simulink model "helicopter_sim"  (R2024b)
settings: Solver=ode4  StartTime=0.0  StopTime=30  FixedStep=ST  RelTol=1e-3
StopFcn:
  | % main rotor flapping restraint
  | if over_flap
  |     warning('MyModel:flapping', '<strong> main rotor blade flapping exceeded limits </strong>');
  | end
  | % tail rotor flapping restraint
  | if over_flap_tr
  |     warning('MyModel:flapping_tr', '<strong> tail rotor blade flapping exceeded limits </strong>');
  | end
  | % main rotor load limit
  | if load_mr
  |     warning('MyModel:load_mr', '<strong> main rotor load limit reached </strong>');
  | end
  | % main rotor power limit
  | if power_mr
  |     warning('MyModel:power_mr', '<strong> transmission maximum power rating reached </strong>');
  | end
  | % main rotor blade stall
  | if stall_mr
  |     warning('MyModel:blade_stall', '<strong> main rotor blade stall </strong>');
  | end
  | clear over_flap over_flap_tr load_mr power_mr stall_mr
values from neighbouring files (symbols this model uses):
  a_0 = [ 0 0 0 ]'*pi/180    [parameters.m]    (also in trim.m = [ flap_ss(1) flap_ss(2) flap_ss(3) ]')
  a_hs = 6    [parameters.m]
  a_vs = 6    [parameters.m]
  AKBETA = 0    [parameters.m]
  AKONE = 0    [parameters.m]
  AKONETR = tan(30*(pi/180))    [parameters.m]
  alpha_stall = 15    [parameters.m]
  AOP = 0    [parameters.m]
  AOPTR = 0    [parameters.m]
  AR_hs = 4.5    [parameters.m]
  AR_vs = 1.8    [parameters.m]
  ASLOPE = 6    [parameters.m]
  ASLOPETR = 6    [parameters.m]
  BLADES = 4    [parameters.m]
  BLADESTR = 3    [parameters.m]
  BLCG = 0    [parameters.m]
  BLHS = 0    [parameters.m]
  BLMR = 0    [parameters.m]
  BLRPF = 0    [parameters.m]
  BLTR = -1.8*Ft_m    (= -0.54864)    [parameters.m]
  BLVS = 0    [parameters.m]
  CD_f = [1.774 0.2043 7]    [parameters.m]
  CD_mr = [0.0107 -0.151 1.72]    [parameters.m]
  CD_tr = [ 0.0107 -0.151 1.72 ]    [parameters.m]
  chi_mr = 1    [parameters.m]
  chi_tr = 1    [parameters.m]
  CHORD = 2*Ft_m    (= 0.6096)    [parameters.m]
  CHORDTR = 1*Ft_m    (= 0.3048)    [parameters.m]
  CL_f = [-0.4279 10.33]    [parameters.m]
  CL_max_hs = 1.2    [parameters.m]
  CL_max_vs = 1.2    [parameters.m]
  CLL_f = [0.0696 6.336]    [parameters.m]
  CM_f = [-4.4961 49.522]    [parameters.m]
  CN_f = [0.0396 -21.699]    [parameters.m]
  CY_f = [-0.0359 -16.987]    [parameters.m]
  D = zeros(9,4)    [linearization.m]
  dyn_viscosity = 17.89e-6    (= 1.789e-05)    [parameters.m]
  e_hs = 0.8    [parameters.m]
  e_vs = 0.8    [parameters.m]
  EPSLN = 0.05    [parameters.m]
  euler0 = [ 0 0 0 ]'*pi/180    [parameters.m]    (also in trim.m = [ euler_trim(1)*abs(max_att) euler_trim(2)*abs(max_att) eule)
  fc = [  100*Kn_mps ... (first row only)    [parameters.m]
  GAMMA = 8.1    [parameters.m]
  GAMMATR = 4    [parameters.m]
  href = 0    [parameters.m]
  i_hs = -3*(pi/180)+a0_hs    (= -0.0523598775598)    [parameters.m]
  i_s = 0    [parameters.m]
  i_vs = 0*(pi/180)+a0_vs    (= -0.0872664625997)    [parameters.m]
  Jbeta = 1/3*m_blade*ROTOR^3*(1-EPSLN)^3    (= 3891.86391298)    [parameters.m]
  k_ind = 1    [parameters.m]
  k_ind_tr = 1    [parameters.m]
  kv_tr = 0.8    [parameters.m]
  Lambda_hs = 13*(pi/180)    (= 0.226892802759)    [parameters.m]
  Lambda_vs = 27*(pi/180)    (= 0.471238898038)    [parameters.m]
  lat_cyc_range = [ -15 15 ]    [parameters.m]
  latref = 39.24744998520548    (= 39.2474499852)    [parameters.m]
  lon_cyc_range = [ -15 15 ]    [parameters.m]
  lonref = 9.050782438199448    (= 9.0507824382)    [parameters.m]
  m = 20000*Lb_Kg    (= 9071.84)    [parameters.m]
  m_blade = 0.372*Slug_Kg/Ft_m    (= 17.8114564173)    [parameters.m]
  max_flap_mr = 20*pi/180    (= 0.349065850399)    [parameters.m]
  max_flap_tr = 20*pi/180    (= 0.349065850399)    [parameters.m]
  max_load = 3*m*9.81    (= 266984.2512)    [parameters.m]
  mode = 0    [linearization.m]    (also in parameters.m; trim.m)
  mr_coll_range = [   0 25 ]    [parameters.m]
  OMEGA = 206.9*(pi/30)    (= 21.6665173343)    [parameters.m]
  omega0 = [ 0 0 0 ]'    [parameters.m]
  OMEGATR = 954.93*(pi/30)    (= 100.000035756)    [parameters.m]
  pilot_trim = [ x(1); x(2); x(3); x(4) ]    [trim.m]
  rated_power = 4170*hp_W    (= 3109569)    [parameters.m]
  ROTOR = 30*Ft_m    (= 9.144)    [parameters.m]
  ROTORTR = 6.5*Ft_m    (= 1.9812)    [parameters.m]
  S_hs = 18*(Ft_m^2)    (= 1.67225472)    [parameters.m]
  S_vs = 33*(Ft_m^2)    (= 3.06580032)    [parameters.m]
  ST = 0.001    [parameters.m]
  STACG = 24.4*Ft_m    (= 7.43712)    [parameters.m]
  STAHS = 57.4*Ft_m    (= 17.49552)    [parameters.m]
  STAMR = 23.9*Ft_m    (= 7.28472)    [parameters.m]
  STARPF = 23.9*Ft_m    (= 7.28472)    [parameters.m]
  STATR = 61.4*Ft_m    (= 18.71472)    [parameters.m]
  STAVS = 59.4*Ft_m    (= 18.10512)    [parameters.m]
  THETT = -10*(pi/180)    (= -0.174532925199)    [parameters.m]
  THETTTR = -5*(pi/180)    (= -0.0872664625997)    [parameters.m]
  tr_coll_range = [   0 20 ]    [parameters.m]
  Ttrb = [ 1 0 0; 0 0 1; 0 -1 0]    [parameters.m]
  V0 = eul2rotm(euler0','XYZ')'*[ fc(1) fc(2) fc(3) ]'    [parameters.m]    (also in trim.m)
  wind_rate = [ 0 0 0 ]'    [parameters.m]
  wind_velocity_e = [ 0 0 0 ]'    [parameters.m]
  WLCG = 9.2*Ft_m    (= 2.80416)    [parameters.m]
  WLHS = 7.7*Ft_m    (= 2.34696)    [parameters.m]
  WLMR = 16.7*Ft_m    (= 5.09016)    [parameters.m]
  WLRPF = 12.2*Ft_m    (= 3.71856)    [parameters.m]
  WLTR = 15.2*Ft_m    (= 4.63296)    [parameters.m]
  WLVS = 12.2*Ft_m    (= 3.71856)    [parameters.m]
  Xe_0 = [ 16404 0 -1000 ]'*Ft_m    [parameters.m]
undefined symbols (not defined in the file or in its folder): Earth, rad, s, WGS84
libraries: simulink x4, aerolibanimutils x2, aerolibsim3d x2, sim3dlib x1, aerolibconvert2 x1, shared6dof x1, aerolibtransform2 x1, aerolibatmos2 x1
(part 1 of 3)
settings Model: Creator=fra62  LastModifiedBy=fra62

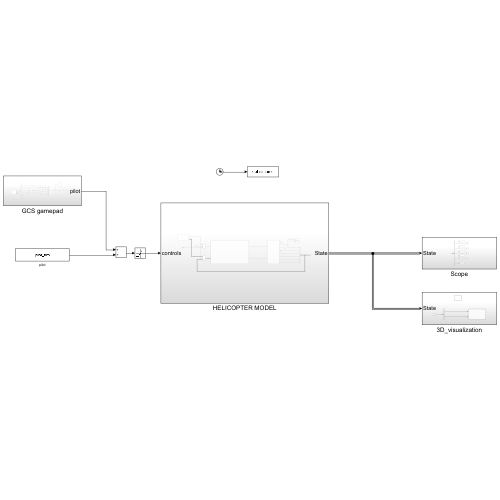
[thumbnail: Simulink's stored preview of the top-level diagram]
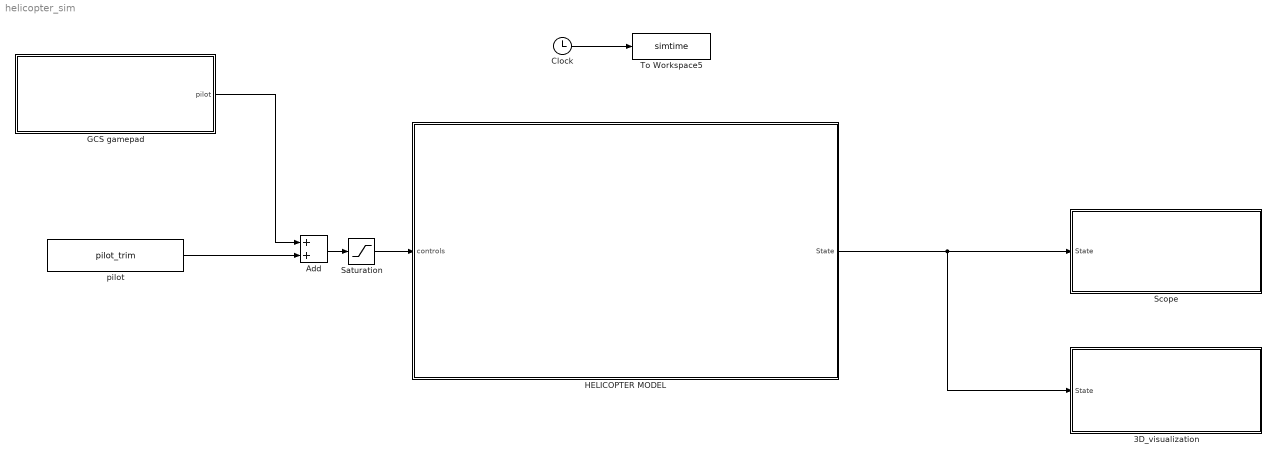
== system helicopter_sim ==
  3D_visualization : Subsystem
  Add : Sum
  Clock : Clock
  GCS gamepad : Subsystem
  HELICOPTER MODEL : Subsystem
  Saturation : Saturate  UpperLimit=1  LowerLimit=-1
  Scope : Subsystem
  To Workspace5 : ToWorkspace  VariableName=simtime  SampleTime=-1
  pilot : Constant  Value=pilot_trim
  wires:
  GCS gamepad/1(pilot) -> Add/1
  pilot/1 -> Add/2
  Saturation/1 -> HELICOPTER MODEL/1(controls)
  Add/1 -> Saturation/1
  Clock/1 -> To Workspace5/1
  HELICOPTER MODEL/1(State) -> 3D_visualization/1(State), Scope/1(State)

== system helicopter_sim/3D_visualization ==
  State : Inport
  Bus Selector : BusSelector  OutputSignals=NED,Euler
  Simulation Pace : aerolibanimutils/Simulation Pace  SimulationPace=1  SleepMode=Auto  OutputPaceError=off  SampleTime=ST
  UNREAL ENGINE 3D SCENE : Subsystem
  wires:
  State/1 -> Bus Selector/1
  Bus Selector/1 -> UNREAL ENGINE 3D SCENE/1(Xe)  "<NED>"
  Bus Selector/2 -> UNREAL ENGINE 3D SCENE/2(euler)  "<Euler>"

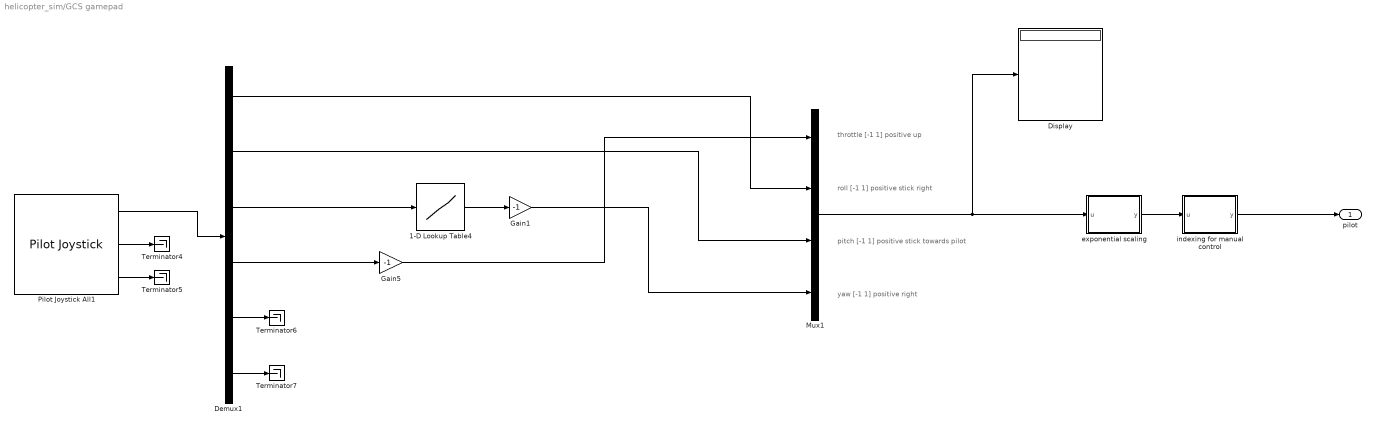
== system helicopter_sim/GCS gamepad ==
  note: yaw [-1 1] positive right
  note: throttle [-1 1] positive up
  note: pitch [-1 1] positive stick towards pilot
  note: roll [-1 1] positive stick right
  " exponential scaling " : MATLAB Function  TreatAsAtomicUnit=on
  1-D Lookup Table4 : Lookup_n-D  NumberOfTableDimensions=1  BreakpointsForDimension1=[0 1]  Table=[-1 1]  InternalRulePriority=Speed  RndMeth=Simplest
  Demux1 : Demux  Outputs=6
  Display : Display
  Gain1 : Gain  Gain=-1
  Gain5 : Gain  Gain=-1
  Mux1 : Mux
  Pilot Joystick All1 : aerolibanimutils/Pilot Joystick  JoystickID=Joystick1  OutputConfiguration=AllOutputs  SampleTime=ST
      settings: LibrarySourceBlock=aerolibanimutils/Pilot Joystick All
  Terminator{4..7} (4 alike) : Terminator
  indexing for manual control : MATLAB Function  TreatAsAtomicUnit=on
  pilot : Outport
  wires:
  Gain5/1 -> Mux1/1
  Demux1/1 -> Mux1/2
  Pilot Joystick All1/3 -> Terminator5/1
  Mux1/1 -> Display/1, " exponential scaling "/1(u)
  Demux1/5 -> Terminator6/1
  Demux1/2 -> Mux1/3
  Pilot Joystick All1/2 -> Terminator4/1
  Demux1/4 -> Gain5/1
  Demux1/3 -> 1-D Lookup Table4/1
  1-D Lookup Table4/1 -> Gain1/1
  Demux1/6 -> Terminator7/1
  Pilot Joystick All1/1 -> Demux1/1
  Gain1/1 -> Mux1/4
  " exponential scaling "/1(y) -> indexing for manual control/1(u)
  indexing for manual control/1(y) -> pilot/1

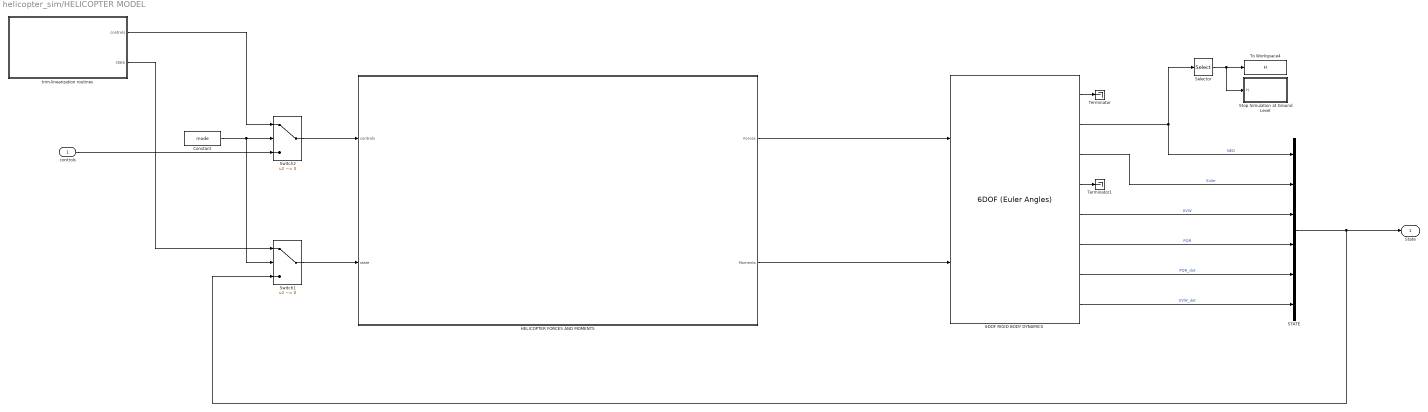
== system helicopter_sim/HELICOPTER MODEL ==
  controls : Inport
  6DOF RIGID BODY DYNAMICS : shared6dof/6DOF (Euler Angles)  units=Metric (MKS)  mtype=Fixed  rep=Euler Angles  xme_0=Xe_0  Vm_0=V0  eul_0=euler0  pm_0=omega0  mass_0=m  mass_e=0.5  mass_f=2.0  inertia=inertia  inertia_e=eye(3)  inertia_f=2*eye(3)  k_quat=1.0  vre_flag=on  abi_flag=off  aMode=0  xme_statename=''  Vm_statename=''  eul_statename=''  quat_statename=''  pm_statename=''  mass_statename=''
  Constant : Constant  Value=mode
  HELICOPTER FORCES AND MOMENTS : Subsystem
  STATE : BusCreator  Inputs=6
  Selector : Selector  InputPortWidth=3  IndexOptions=Index vector (dialog)  Indices=[3]  OutputSizes=1
  Stop Simulation at Ground Level : Subsystem
  Switch1 : Switch  Criteria=u2 ~= 0  SaturateOnIntegerOverflow=off  InputSameDT=off
  Switch2 : Switch  Criteria=u2 ~= 0  SaturateOnIntegerOverflow=off  InputSameDT=off
  Terminator : Terminator
  Terminator1 : Terminator
  To Workspace4 : ToWorkspace  VariableName=H  SampleTime=-1
  trim-linearization routines : Subsystem
  State : Outport
  wires:
  STATE/1 -> State/1, Switch1/3
  6DOF RIGID BODY DYNAMICS/6 -> STATE/4  "PQR"
  6DOF RIGID BODY DYNAMICS/3 -> STATE/2  "Euler"
  6DOF RIGID BODY DYNAMICS/5 -> STATE/3  "UVW"
  6DOF RIGID BODY DYNAMICS/1 -> Terminator/1
  6DOF RIGID BODY DYNAMICS/4 -> Terminator1/1
  6DOF RIGID BODY DYNAMICS/2 -> Selector/1, STATE/1  "NED"
  6DOF RIGID BODY DYNAMICS/8 -> STATE/6  "UVW_dot"
  controls/1 -> Switch2/3
  6DOF RIGID BODY DYNAMICS/7 -> STATE/5  "PQR_dot"
  Switch2/1 -> HELICOPTER FORCES AND MOMENTS/1(controls)
  Switch1/1 -> HELICOPTER FORCES AND MOMENTS/2(state)
  trim-linearization routines/2(state) -> Switch1/1
  trim-linearization routines/1(controls) -> Switch2/1
  Constant/1 -> Switch1/2, Switch2/2
  HELICOPTER FORCES AND MOMENTS/1(Forces) -> 6DOF RIGID BODY DYNAMICS/1
  HELICOPTER FORCES AND MOMENTS/2(Moments) -> 6DOF RIGID BODY DYNAMICS/2
  Selector/1 -> To Workspace4/1, Stop Simulation at Ground Level/1(H)

== system helicopter_sim/Scope ==
  State : Inport
  Bus Selector : BusSelector  OutputSignals=UVW,PQR,NED,Euler,UVW_dot
  Gain : Gain  Gain=180/pi
  To Workspace1 : ToWorkspace  VariableName=UVW  SampleTime=-1
      settings: Save2DSignal=2-D array (concatenate along first dimension)
  To Workspace2 : ToWorkspace  VariableName=Euler  SampleTime=-1
      settings: Save2DSignal=2-D array (concatenate along first dimension)
  To Workspace3 : ToWorkspace  VariableName=PQR  SampleTime=-1
      settings: Save2DSignal=2-D array (concatenate along first dimension)
  To Workspace5 : ToWorkspace  VariableName=NED  SampleTime=-1
      settings: Save2DSignal=2-D array (concatenate along first dimension)
  To Workspace8 : ToWorkspace  VariableName=UVW_dot  SampleTime=-1
      settings: Save2DSignal=2-D array (concatenate along first dimension)
  attitude : Scope
  position : Scope
  rates : Scope
  velocity : Scope
  wires:
  State/1 -> Bus Selector/1
  Bus Selector/1 -> To Workspace1/1, velocity/1  "<UVW>"
  Bus Selector/2 -> To Workspace3/1, rates/1  "<PQR>"
  Bus Selector/3 -> To Workspace5/1, position/1  "<NED>"
  Bus Selector/4 -> To Workspace2/1, Gain/1  "<Euler>"
  Gain/1 -> attitude/1
  Bus Selector/5 -> To Workspace8/1  "<UVW_dot>"

== system helicopter_sim/3D_visualization/UNREAL ENGINE 3D SCENE ==
  Xe : Inport
  euler : Inport  Port=2
  Constant : Constant  Value=OMEGA
  Constant1 : Constant  Value=OMEGATR
  Simulation 3D Light Helicopter Pack : aerolibsim3d/Simulation 3D Light Helicopter Pack  Engine_T=off  Engine_R=off  Rotor1_T=off  Rotor1_R=on  Rotor2_T=off  Rotor2_R=on  Sensor1_T=off  Sensor1_R=off  Sensor2_T=off  Sensor2_R=off  GeoRadioButton=NED  AdjustForCesium=off  Heading0=90
  Simulation 3D Rotorcraft : aerolibsim3d/Simulation 3D Rotorcraft  Priority=-1  Mesh=Light helicopter  MeshPath=/MathWorksAerospaceContent/Vehicles/Rotorcraft/Helicopter/Mesh/SK_Helicopter.SK_Helicopter  MeshPathLight=/MathWorksAerospaceContent/Vehicles/Rotorcraft/LightHelicopter/Mesh/SK_LightHelicopter.SK_LightHelicopter  MeshPathMulti=/MathWorksAerospaceContent/Vehicles/Rotorcraft/Multirotor/Mesh/SK_Quadcopter.SK_Quadcopter  AircraftColor=Red  ActorName=helicopter  Translation=[Xe_0(1) Xe_0(2) Xe_0(3);zeros(5,3)]  Rotation=zeros(6, 3)  ScaleInputPort=Dialog  Scale=[1 1 1]  InitialScale=[1 1 1]  IsGHSensorEnabled=off  AreGHRaysVisible=off  IsOutputReshapeEnabled=off  GHRayLength=1524  GHBodyOffset=1.169  GHFrontTireRadius=0.196  GHLeftTireRadius=0.203  GHRightTireRadius=0.203  GHContactLocation1=[1.47 -1.04 1.169]  GHContactLocation2=[-1.24 -1.04 1.169]  GHContactLocation3=[-1.24 1.04 1.169]  GHContactLocation4=[1.47 1.04 1.169]  WoWSensorTolerance=0.05  LightsConfig=Automatic lights  LandingLightIntensity=300000  LandingLightConeAngle=15  LandingLightColor=[1 1 1]  HelicopterLeftLandingLightLocation=[0 0 0]  HelicopterLeftLandingLightOrientation=[0 0 0]  NoseLightIntensity=150000  NoseLightConeAngle=36  HelicopterNoseLightLocation=[0 0 0]  HelicopterNoseLightOrientation=[0 0 0]  NavLightIntensity=500  PositionLightIntensity=500  StrobeLightIntensity=5000  StrobeLightColor=[1 1 1]  StrobePeriod=1.5  StrobePulseWidth=6  BeaconLightIntensity=4000  BeaconLightColor=[1 0 0]  BeaconPeriod=1.5  BeaconPulseWidth=10  SampleTime=-1  ActorType=SimulinkVehicle  ID=C  aMode=0  ActorTag=helicopter
  Simulation 3D Scene Configuration1 : sim3dlib/Simulation 3D Scene Configuration  Priority=0  ProjectFormat=Default Scenes  SceneDesc=Airport  ProjectName=C:\Program Files\MATLAB\R2024b\toolbox\shared\sim3d_projects\automotive_project_windows\UE\WindowsNoEditor\VehicleSimulation.exe  ScenePath=/Game/Maps/HwStrght  EnableOpenDRIVE=off  vehTagList={'Custom';'Prouty example helicopter (medium size utility)';'Scene Origin';'SimulinkVehicle1';'helicopter'}  vehTag=helicopter  FreeCameraInitialTranslation=[-6, 0, 2]  FreeCameraDefaultInitialTranslation=[-6, 0, 2]  FreeCameraInitialRotation=[0, -15, 0]  FreeCameraDefaultInitialRotation=[0, -15, 0]  OpVisEn=off  Ts=.03  EnableWindow=on  EnableRemoteAccess=off  EnableWeather=off  SunAzimuth=90  SunAltitude=40.0  EnableGeospatialSun=off  Latitude=0  Longitude=0  Date=2023-01-01  Time=10:30:00  GeoTimeZone=-5.0  SunDaylightSaving=off  wind=1  clouds=10  EnableVolumetricClouds=off  CloudCoverage=0  CloudAltitude=6  fog=0  rain=0  RaindropsEffect=off  SnowDensity=0  EnableGeospatial=off  UseTrueOrigin=off  OriginHeight=200  OriginLatitude=40.744652  OriginLongitude=-73.988864  MapStyle=Aerial  AdditionalAssetIDs=[]  UseAdvancedSunSky=off  SolarTime=11  TimeZone=-5  Day=21  Month=9  Year=2022  UseDaylightSavingTime=on  DSTStartDay=10  DSTStartMonth=3  DSTEndDay=3  DSTEndMonth=11  DSTSwitchHour=2  sensorTag=MainCamera2  sensorId=2  sensorName=MainCamera2  mountLoc=Origin  offsetFlag=off  tmountOffset=[0, 0, 0]  rmountOffset=[0, 0, 0]  HorizontalResolution=1280  VerticalResolution=720  HorizontalFOV=60  mountPoint=[0 0 0]  mountOrientation=[0 0 0]  aMode=0  ID=2  GeoTrigger=Inactive
      settings: LibrarySourceBlock=aerolibsim3d/Simulation 3D Scene Configuration
  Subsystem : Subsystem
  wires:
  Constant1/1 -> Subsystem/2(SpeedT)
  Constant/1 -> Subsystem/1(SpeedM)
  Subsystem/2(Position Blade 2) -> Simulation 3D Light Helicopter Pack/4
  Subsystem/1(Position Blade1) -> Simulation 3D Light Helicopter Pack/3
  Simulation 3D Light Helicopter Pack/1 -> Simulation 3D Rotorcraft/1
  Simulation 3D Light Helicopter Pack/2 -> Simulation 3D Rotorcraft/2
  euler/1 -> Simulation 3D Light Helicopter Pack/2
  Xe/1 -> Simulation 3D Light Helicopter Pack/1

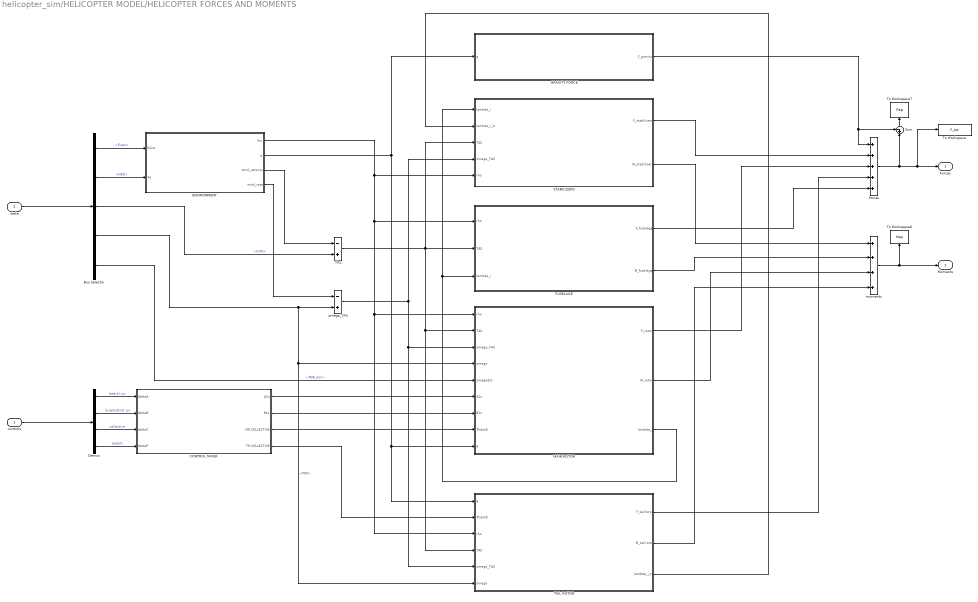
== system helicopter_sim/HELICOPTER MODEL/HELICOPTER FORCES AND MOMENTS ==
  controls : Inport
  state : Inport  Port=2
  Bus Selector : BusSelector  OutputSignals=Euler,NED,UVW,PQR,PQR_dot
  CONTROL MIXER : Subsystem
  Demux : Demux
  ENVIRONMENT : Subsystem
  "FUSELAGE " : Subsystem
  "GRAVITY FORCE " : Subsystem
  MAIN ROTOR : Subsystem
  "STABILIZERS " : Subsystem
  Sum : Sum  Inputs=-+|
  "TAIL ROTOR " : Subsystem
  TAS : Sum  Inputs=-+
  To Workspace : ToWorkspace  VariableName=F_tot  SampleTime=-1
  To Workspace6 : ToWorkspace  VariableName=Map  SampleTime=-1
  To Workspace7 : ToWorkspace  VariableName=Fap  SampleTime=-1
  forces : Sum  Inputs=+++++
  moments : Sum  Inputs=++++
  omega_TAS : Sum  Inputs=-+
  Forces : Outport
  Moments : Outport  Port=2
  wires:
  Demux/1 -> CONTROL MIXER/1(deltaA)  "lateral cyc"
  Bus Selector/4 -> MAIN ROTOR/4(omega), "TAIL ROTOR "/6(omega), omega_TAS/2  "<PQR>"
  forces/1 -> To Workspace/1, Forces/1, Sum/2
  omega_TAS/1 -> "STABILIZERS "/4(omega_TAS), MAIN ROTOR/3(omega_TAS), "TAIL ROTOR "/5(omega_TAS)
  Bus Selector/5 -> MAIN ROTOR/5(omegadot)  "<PQR_dot>"
  Sum/1 -> To Workspace7/1
  Bus Selector/3 -> TAS/2  "<UVW>"
  Demux/2 -> CONTROL MIXER/2(deltaB)  "longitudinal cyc"
  MAIN ROTOR/2(M_rotor) -> moments/3
  moments/1 -> Moments/1, To Workspace6/1
  Demux/3 -> CONTROL MIXER/3(deltaC)  "collective"
  ENVIRONMENT/1(rho) -> "STABILIZERS "/5(rho), MAIN ROTOR/1(rho), "TAIL ROTOR "/3(rho), "FUSELAGE "/1(rho)
  CONTROL MIXER/3(MR COLLECTIVE) -> MAIN ROTOR/8(Theta0)
  ENVIRONMENT/2(g) -> "GRAVITY FORCE "/1(g), MAIN ROTOR/9(g), "TAIL ROTOR "/1(g)
  MAIN ROTOR/1(F_rotor) -> forces/3
  CONTROL MIXER/2(B1s) -> MAIN ROTOR/7(B1s)
  "TAIL ROTOR "/2(M_tailrotor) -> moments/4
  "STABILIZERS "/2(M_stabilizers) -> moments/1
  CONTROL MIXER/4(TR COLLECTIVE) -> "TAIL ROTOR "/2(Theta0)
  "TAIL ROTOR "/1(F_tailrotor) -> forces/4
  ENVIRONMENT/3(wind_velocity) -> TAS/1
  CONTROL MIXER/1(A1s) -> MAIN ROTOR/6(A1s)
  "FUSELAGE "/1(F_fuselage) -> forces/5
  "FUSELAGE "/2(M_fuselage) -> moments/2
  TAS/1 -> "STABILIZERS "/3(TAS), "FUSELAGE "/2(TAS), MAIN ROTOR/2(TAS), "TAIL ROTOR "/4(TAS)
  "GRAVITY FORCE "/1(F_gravity) -> forces/1, Sum/1
  Bus Selector/1 -> ENVIRONMENT/1(Euler)  "<Euler>"
  "STABILIZERS "/1(F_stabilizers) -> forces/2
  ENVIRONMENT/4(wind_rate) -> omega_TAS/1
  Demux/4 -> CONTROL MIXER/4(deltaP)  "pedals"
  controls/1 -> Demux/1
  MAIN ROTOR/3(lambda_i) -> "STABILIZERS "/1(lambda_i), "FUSELAGE "/3(lambda_i)
  "TAIL ROTOR "/3(lambda_i_tr) -> "STABILIZERS "/2(lambda_i_tr)
  state/1 -> Bus Selector/1
  Bus Selector/2 -> ENVIRONMENT/2(Xe)  "<NED>"

== system helicopter_sim/HELICOPTER MODEL/Stop Simulation at Ground Level ==
  H : Inport
  Compare To Constant : simulink/Logic and Bit Operations/Compare To Constant  relop=>  const=0.1  OutDataTypeStr=boolean
  MATLAB Function : MATLAB Function  TreatAsAtomicUnit=on
  Stop Simulation : Stop
  wires:
  H/1 -> Compare To Constant/1
  Compare To Constant/1 -> MATLAB Function/1(u), Stop Simulation/1

== system helicopter_sim/HELICOPTER MODEL/trim-linearization routines ==
  Constant : Constant  Value=mode
  Constant1 : Constant  Value=pilot_trim
  LINEARIZATION : Subsystem
  Multiport Switch1 : MultiPortSwitch  Inputs=2  DiagnosticForDefault=None  SaturateOnIntegerOverflow=off  InputSameDT=off
  TRIM : Subsystem
  controls : Outport
  state : Outport  Port=2
  wires:
  Multiport Switch1/1 -> state/1
  TRIM/1(state) -> Multiport Switch1/2
  LINEARIZATION/1(state) -> Multiport Switch1/3
  Constant/1 -> Multiport Switch1/1
  Constant1/1 -> controls/1

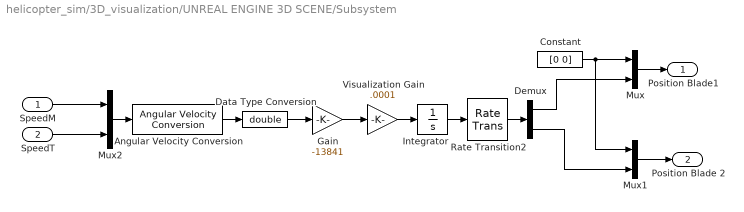
== system helicopter_sim/3D_visualization/UNREAL ENGINE 3D SCENE/Subsystem ==
  SpeedM : Inport
  SpeedT : Inport  Port=2
  Angular Velocity Conversion : aerolibconvert2/Angular Velocity Conversion  IU=rad/s  OU=rpm
  Constant : Constant  Value=[0 0]  VectorParams1D=off
  Data Type Conversion : DataTypeConversion  OutDataTypeStr=double  SaturateOnIntegerOverflow=off  RndMeth=Floor
  Demux : Demux  Outputs=2
  Gain : Gain  Gain=-13841
  Integrator : Integrator  InitialCondition="[.1  .1]"  WrapState=on  WrappedStateUpperValue=2*pi  WrappedStateLowerValue=-2*pi
  Mux : Mux  Inputs=2
  Mux1 : Mux  Inputs=2
  Mux2 : Mux  Inputs=2
  Rate Transition2 : RateTransition
  Visualization Gain : Gain  Gain=.0001
  Position Blade1 : Outport  VectorParamsAs1DForOutWhenUnconnected=off
  Position Blade 2 : Outport  Port=2  VectorParamsAs1DForOutWhenUnconnected=off
  wires:
  Demux/2 -> Mux1/2
  Visualization Gain/1 -> Integrator/1
  Constant/1 -> Mux1/1, Mux/1
  Mux1/1 -> Position Blade 2/1
  Data Type Conversion/1 -> Gain/1
  Integrator/1 -> Rate Transition2/1
  Mux/1 -> Position Blade1/1
  Gain/1 -> Visualization Gain/1
  Demux/1 -> Mux/2
  Mux2/1 -> Angular Velocity Conversion/1
  Rate Transition2/1 -> Demux/1
  SpeedM/1 -> Mux2/1
  SpeedT/1 -> Mux2/2
  Angular Velocity Conversion/1 -> Data Type Conversion/1

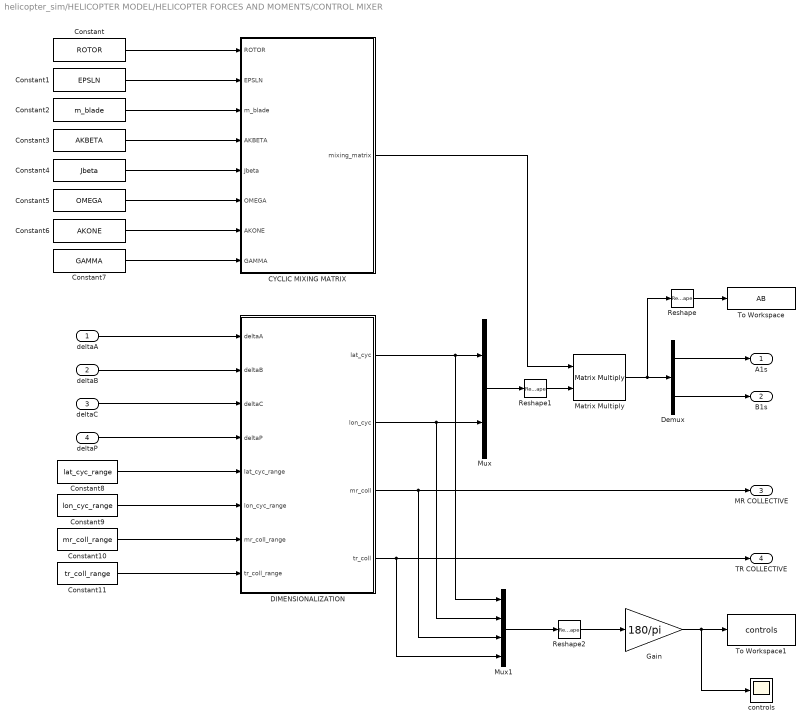
== system helicopter_sim/HELICOPTER MODEL/HELICOPTER FORCES AND MOMENTS/CONTROL MIXER ==
  deltaA : Inport
  deltaB : Inport  Port=2
  deltaC : Inport  Port=3
  deltaP : Inport  Port=4
  CYCLIC MIXING MATRIX : MATLAB Function  TreatAsAtomicUnit=on
  Constant : Constant  Value=ROTOR
  Constant1 : Constant  Value=EPSLN
  Constant10 : Constant  Value=mr_coll_range
  Constant11 : Constant  Value=tr_coll_range
  Constant2 : Constant  Value=m_blade
  Constant3 : Constant  Value=AKBETA
  Constant4 : Constant  Value=Jbeta
  Constant5 : Constant  Value=OMEGA
  Constant6 : Constant  Value=AKONE
  Constant7 : Constant  Value=GAMMA
  Constant8 : Constant  Value=lat_cyc_range
  Constant9 : Constant  Value=lon_cyc_range
  DIMENSIONALIZATION : MATLAB Function  TreatAsAtomicUnit=on
  Demux : Demux  Outputs=2
  Gain : Gain  Gain=180/pi
  Matrix Multiply : Product  Multiplication=Matrix(*)
  Mux : Mux  Inputs=2
  Mux1 : Mux
  Reshape : Reshape  OutputDimensionality=Column vector (2-D)
  Reshape1 : Reshape  OutputDimensionality=Column vector (2-D)
  Reshape2 : Reshape  OutputDimensionality=Column vector (2-D)
  To Workspace : ToWorkspace  VariableName=AB  SampleTime=-1
  To Workspace1 : ToWorkspace  VariableName=controls  SampleTime=-1
  controls : Scope
  A1s : Outport
  B1s : Outport  Port=2
  MR COLLECTIVE : Outport  Port=3
  TR COLLECTIVE : Outport  Port=4
  wires:
  Demux/2 -> B1s/1
  Mux/1 -> Reshape1/1
  Demux/1 -> A1s/1
  CYCLIC MIXING MATRIX/1(mixing_matrix) -> Matrix Multiply/1
  Constant/1 -> CYCLIC MIXING MATRIX/1(ROTOR)
  Constant1/1 -> CYCLIC MIXING MATRIX/2(EPSLN)
  Constant2/1 -> CYCLIC MIXING MATRIX/3(m_blade)
  Constant3/1 -> CYCLIC MIXING MATRIX/4(AKBETA)
  Constant4/1 -> CYCLIC MIXING MATRIX/5(Jbeta)
  Constant5/1 -> CYCLIC MIXING MATRIX/6(OMEGA)
  Constant6/1 -> CYCLIC MIXING MATRIX/7(AKONE)
  Constant7/1 -> CYCLIC MIXING MATRIX/8(GAMMA)
  DIMENSIONALIZATION/1(lat_cyc) -> Mux1/1, Mux/1
  DIMENSIONALIZATION/2(lon_cyc) -> Mux1/2, Mux/2
  deltaP/1 -> DIMENSIONALIZATION/4(deltaP)
  deltaC/1 -> DIMENSIONALIZATION/3(deltaC)
  deltaB/1 -> DIMENSIONALIZATION/2(deltaB)
  deltaA/1 -> DIMENSIONALIZATION/1(deltaA)
  DIMENSIONALIZATION/3(mr_coll) -> MR COLLECTIVE/1, Mux1/3
  DIMENSIONALIZATION/4(tr_coll) -> TR COLLECTIVE/1, Mux1/4
  Constant8/1 -> DIMENSIONALIZATION/5(lat_cyc_range)
  Constant9/1 -> DIMENSIONALIZATION/6(lon_cyc_range)
  Constant10/1 -> DIMENSIONALIZATION/7(mr_coll_range)
  Constant11/1 -> DIMENSIONALIZATION/8(tr_coll_range)
  Reshape1/1 -> Matrix Multiply/2
  Reshape/1 -> To Workspace/1
  Matrix Multiply/1 -> Reshape/1, Demux/1
  Gain/1 -> controls/1, To Workspace1/1
  Reshape2/1 -> Gain/1
  Mux1/1 -> Reshape2/1

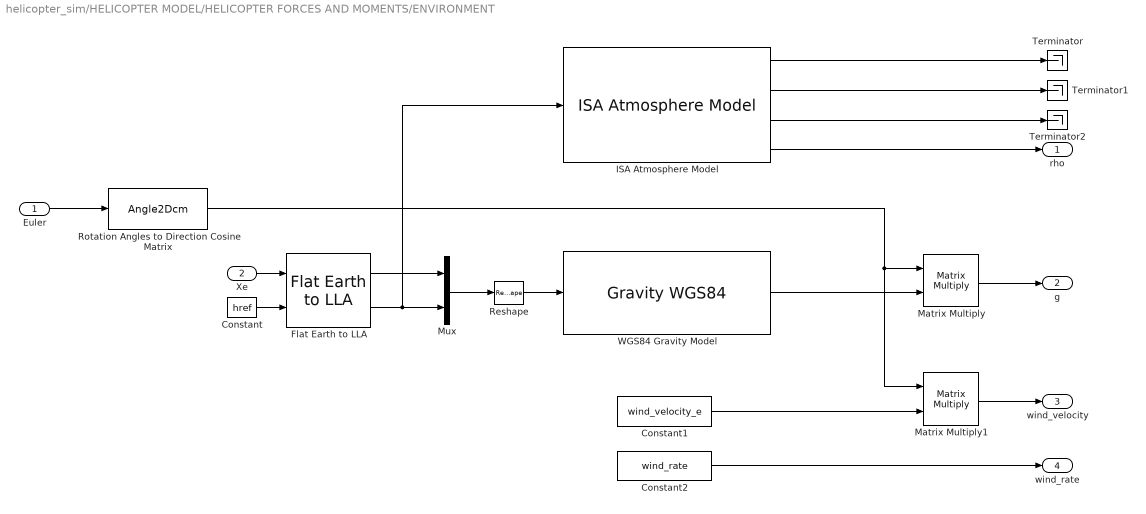
== system helicopter_sim/HELICOPTER MODEL/HELICOPTER FORCES AND MOMENTS/ENVIRONMENT ==
  Euler : Inport
  Xe : Inport  Port=2
  Constant : Constant  Value=href
  Constant1 : Constant  Value=wind_velocity_e
  Constant2 : Constant  Value=wind_rate
  Flat Earth to LLA : aerolibtransform2/Flat Earth to LLA  units=Metric (MKS)  ptype=Earth (WGS84)  F=1/298.257223563  R=6378137  refPosPort=off  LL0=[latref lonref]  psi=0
  ISA Atmosphere Model : aerolibatmos2/ISA Atmosphere Model  useExtended=off  action=Warning  custom=off  viscosityOut=off  g=9.80665  gamma=1.4  R=287.0531  L=0.0065  h_trop=11000  h_strat=20000  rho0=1.225  P0=101325  T0=288.15  h0=0  S=110.4  Tref=273.15  muref=1.716e-5
  Matrix Multiply : Product  Multiplication=Matrix(*)
  Matrix Multiply1 : Product  Multiplication=Matrix(*)
  Mux : Mux  Inputs=[2 1]
  Reshape : Reshape
  Rotation Angles to Direction Cosine Matrix : Angle2Dcm  rotationOrder=XYZ
      settings: AttributesFormatString=Rotation Order: %<rotationOrder>
  Terminator : Terminator
  Terminator1 : Terminator
  Terminator2 : Terminator
  "WGS84 Gravity Model  " : GravityWGS84
  rho : Outport
  g : Outport  Port=2
  wind_velocity : Outport  Port=3
  wind_rate : Outport  Port=4
  wires:
  Mux/1 -> Reshape/1
  ISA Atmosphere Model/2 -> Terminator1/1
  Reshape/1 -> "WGS84 Gravity Model  "/1
  Flat Earth to LLA/2 -> ISA Atmosphere Model/1, Mux/2
  Matrix Multiply/1 -> g/1
  Euler/1 -> Rotation Angles to Direction Cosine Matrix/1
  ISA Atmosphere Model/4 -> rho/1
  Flat Earth to LLA/1 -> Mux/1
  Constant2/1 -> wind_rate/1
  Constant/1 -> Flat Earth to LLA/2
  Xe/1 -> Flat Earth to LLA/1
  Constant1/1 -> Matrix Multiply1/2
  Matrix Multiply1/1 -> wind_velocity/1
  ISA Atmosphere Model/1 -> Terminator/1
  ISA Atmosphere Model/3 -> Terminator2/1
  "WGS84 Gravity Model  "/1 -> Matrix Multiply/2
  Rotation Angles to Direction Cosine Matrix/1 -> Matrix Multiply1/1, Matrix Multiply/1

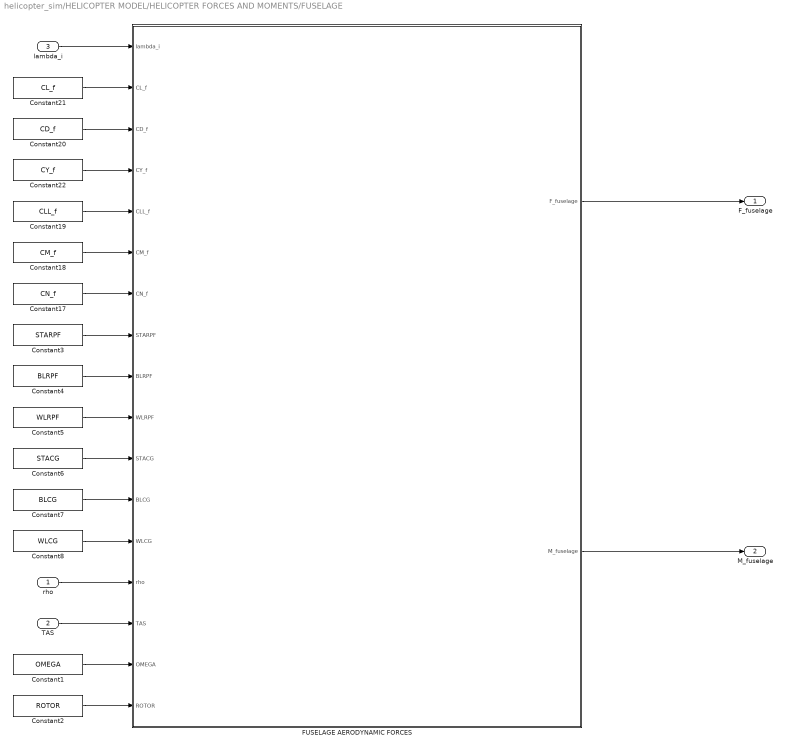
== system helicopter_sim/HELICOPTER MODEL/HELICOPTER FORCES AND MOMENTS/FUSELAGE  ==
  rho : Inport
  TAS : Inport  Port=2
  lambda_i : Inport  Port=3
  Constant1 : Constant  Value=OMEGA
  Constant17 : Constant  Value=CN_f
  Constant18 : Constant  Value=CM_f
  Constant19 : Constant  Value=CLL_f
  Constant2 : Constant  Value=ROTOR
  Constant20 : Constant  Value=CD_f
  Constant21 : Constant  Value=CL_f
  Constant22 : Constant  Value=CY_f
  Constant3 : Constant  Value=STARPF
  Constant4 : Constant  Value=BLRPF
  Constant5 : Constant  Value=WLRPF
  Constant6 : Constant  Value=STACG
  Constant7 : Constant  Value=BLCG
  Constant8 : Constant  Value=WLCG
  FUSELAGE AERODYNAMIC FORCES : MATLAB Function  TreatAsAtomicUnit=on
  F_fuselage : Outport
  M_fuselage : Outport  Port=2
  wires:
  TAS/1 -> FUSELAGE AERODYNAMIC FORCES/15(TAS)
  Constant7/1 -> FUSELAGE AERODYNAMIC FORCES/12(BLCG)
  rho/1 -> FUSELAGE AERODYNAMIC FORCES/14(rho)
  Constant4/1 -> FUSELAGE AERODYNAMIC FORCES/9(BLRPF)
  lambda_i/1 -> FUSELAGE AERODYNAMIC FORCES/1(lambda_i)
  Constant8/1 -> FUSELAGE AERODYNAMIC FORCES/13(WLCG)
  Constant5/1 -> FUSELAGE AERODYNAMIC FORCES/10(WLRPF)
  Constant6/1 -> FUSELAGE AERODYNAMIC FORCES/11(STACG)
  Constant3/1 -> FUSELAGE AERODYNAMIC FORCES/8(STARPF)
  Constant21/1 -> FUSELAGE AERODYNAMIC FORCES/2(CL_f)
  Constant20/1 -> FUSELAGE AERODYNAMIC FORCES/3(CD_f)
  Constant19/1 -> FUSELAGE AERODYNAMIC FORCES/5(CLL_f)
  Constant18/1 -> FUSELAGE AERODYNAMIC FORCES/6(CM_f)
  Constant17/1 -> FUSELAGE AERODYNAMIC FORCES/7(CN_f)
  Constant22/1 -> FUSELAGE AERODYNAMIC FORCES/4(CY_f)
  Constant1/1 -> FUSELAGE AERODYNAMIC FORCES/16(OMEGA)
  Constant2/1 -> FUSELAGE AERODYNAMIC FORCES/17(ROTOR)
  FUSELAGE AERODYNAMIC FORCES/1(F_fuselage) -> F_fuselage/1
  FUSELAGE AERODYNAMIC FORCES/2(M_fuselage) -> M_fuselage/1

== system helicopter_sim/HELICOPTER MODEL/HELICOPTER FORCES AND MOMENTS/GRAVITY FORCE  ==
  g : Inport
  Gain : Gain  Gain=m
  F_gravity : Outport
  wires:
  g/1 -> Gain/1
  Gain/1 -> F_gravity/1

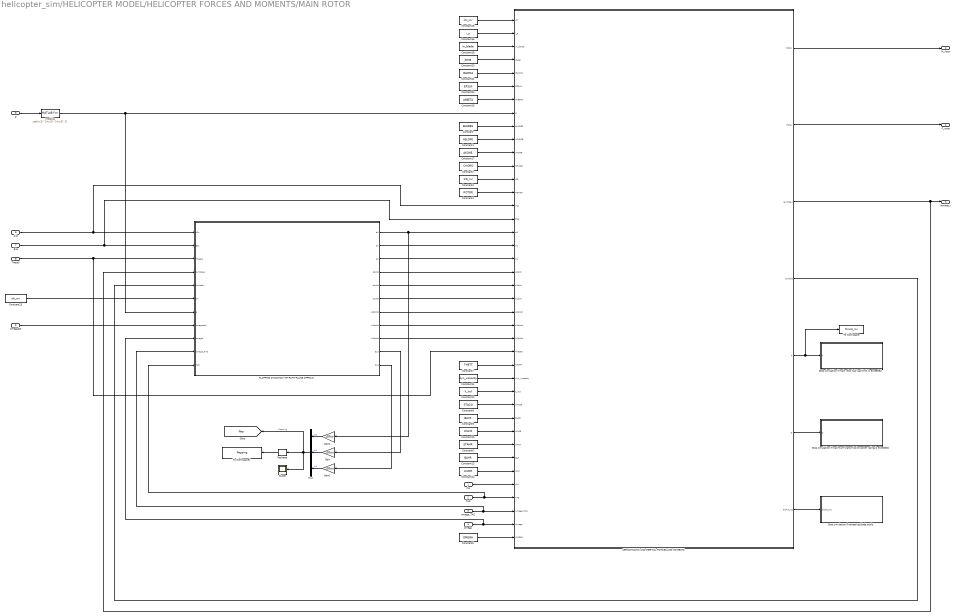
== system helicopter_sim/HELICOPTER MODEL/HELICOPTER FORCES AND MOMENTS/MAIN ROTOR ==
  rho : Inport
  TAS : Inport  Port=2
  omega_TAS : Inport  Port=3
  omega : Inport  Port=4
  omegadot : Inport  Port=5
  A1s : Inport  Port=6
  B1s : Inport  Port=7
  Theta0 : Inport  Port=8
  g : Inport  Port=9
  AERODYNAMIC AND INERTIAL FORCES AND MOMENTS : MATLAB Function  TreatAsAtomicUnit=on
  Constant : Constant  Value=BLADES
  Constant1 : Constant  Value=ASLOPE
  Constant10 : Constant  Value=WLCG
  Constant11 : Constant  Value=dyn_viscosity
  Constant12 : Constant  Value=k_ind
  Constant13 : Constant  Value=BLMR
  Constant14 : Constant  Value=WLMR
  Constant15 : Constant  Value=chi_mr
  Constant16 : Constant  Value=i_s
  Constant17 : Constant  Value=AKONE
  Constant18 : Constant  Value=m_blade
  Constant19 : Constant  Value=AKBETA
  Constant2 : Constant  Value=CHORD
  Constant20 : Constant  Value=Jbeta
  Constant21 : Constant  Value=GAMMA
  Constant22 : Constant  Value=EPSLN
  Constant23 : Constant  Value=chi_mr
  Constant3 : Constant  Value=CD_mr
  Constant4 : Constant  Value=ROTOR
  Constant5 : Constant  Value=OMEGA
  Constant6 : Constant  Value=STAMR
  Constant7 : Constant  Value=THETT
  Constant8 : Constant  Value=STACG
  Constant9 : Constant  Value=BLCG
  FLAPPING DYNAMICS (TIP-PATH-PLANE APPROX) : Subsystem
  Gain : Gain  Gain=180/pi
  Gain1 : Gain  Gain=180/pi
  Gain2 : Gain  Gain=180/pi
  Mux : Mux  Inputs=3
  Reshape : Reshape  OutputDimensionality=Column vector (2-D)
  Scope : Scope
  "Stop simulation if retreating blade stalls " : Subsystem
  Stop simulation if main rotor hub load limit is exceeded : Subsystem
  Stop simulation if maximum transmission power rating is exceeded : Subsystem
  To Workspace : ToWorkspace  VariableName=thrust_mr  SampleTime=-1
  To Workspace1 : ToWorkspace  VariableName=flapping  SampleTime=-1
  "modulus " : MATLABFcn  MATLABFcn=sqrt(u(1)^2+u(2)^2+u(3)^2)
  F_rotor : Outport
  M_rotor : Outport  Port=2
  lambda_i : Outport  Port=3
  tag scope: flap=global
  wires:
  omegadot/1 -> FLAPPING DYNAMICS (TIP-PATH-PLANE APPROX)/8(omegadot)
  FLAPPING DYNAMICS (TIP-PATH-PLANE APPROX)/10(a1s) -> Gain/1
  FLAPPING DYNAMICS (TIP-PATH-PLANE APPROX)/6(b1dot) -> AERODYNAMIC AND INERTIAL FORCES AND MOMENTS/22(b1dot)
  FLAPPING DYNAMICS (TIP-PATH-PLANE APPROX)/2(a1) -> AERODYNAMIC AND INERTIAL FORCES AND MOMENTS/18(a1)
  FLAPPING DYNAMICS (TIP-PATH-PLANE APPROX)/4(a0dot) -> AERODYNAMIC AND INERTIAL FORCES AND MOMENTS/20(a0dot)
  Constant23/1 -> FLAPPING DYNAMICS (TIP-PATH-PLANE APPROX)/6(chi)
  FLAPPING DYNAMICS (TIP-PATH-PLANE APPROX)/8(a1ddot) -> AERODYNAMIC AND INERTIAL FORCES AND MOMENTS/24(a1ddot)
  AERODYNAMIC AND INERTIAL FORCES AND MOMENTS/7(alpha_loc) -> "Stop simulation if retreating blade stalls "/1(alpha_loc)
  FLAPPING DYNAMICS (TIP-PATH-PLANE APPROX)/3(b1) -> AERODYNAMIC AND INERTIAL FORCES AND MOMENTS/19(b1)
  Constant14/1 -> AERODYNAMIC AND INERTIAL FORCES AND MOMENTS/35(WLH)
  g/1 -> "modulus "/1
  Mux/1 -> [flap], Scope/1, Reshape/1  "flapping"
  Gain1/1 -> Mux/3  "b1"
  omega/1 -> AERODYNAMIC AND INERTIAL FORCES AND MOMENTS/39(omega), FLAPPING DYNAMICS (TIP-PATH-PLANE APPROX)/9(omega)
  Constant19/1 -> AERODYNAMIC AND INERTIAL FORCES AND MOMENTS/7(AKBETA)
  AERODYNAMIC AND INERTIAL FORCES AND MOMENTS/1(Mrotor) -> M_rotor/1
  A1s/1 -> FLAPPING DYNAMICS (TIP-PATH-PLANE APPROX)/1(A1s), AERODYNAMIC AND INERTIAL FORCES AND MOMENTS/15(A1s)
  Constant13/1 -> AERODYNAMIC AND INERTIAL FORCES AND MOMENTS/34(BLH)
  Constant10/1 -> AERODYNAMIC AND INERTIAL FORCES AND MOMENTS/32(WLCG)
  Constant7/1 -> AERODYNAMIC AND INERTIAL FORCES AND MOMENTS/27(THETT)
  B1s/1 -> FLAPPING DYNAMICS (TIP-PATH-PLANE APPROX)/2(B1s), AERODYNAMIC AND INERTIAL FORCES AND MOMENTS/16(B1s)
  Gain2/1 -> Mux/1  "a0"
  FLAPPING DYNAMICS (TIP-PATH-PLANE APPROX)/11(b1s) -> Gain1/1
  Reshape/1 -> To Workspace1/1
  Constant17/1 -> AERODYNAMIC AND INERTIAL FORCES AND MOMENTS/11(AKONE)
  Constant9/1 -> AERODYNAMIC AND INERTIAL FORCES AND MOMENTS/31(BLCG)
  TAS/1 -> FLAPPING DYNAMICS (TIP-PATH-PLANE APPROX)/11(TAS), AERODYNAMIC AND INERTIAL FORCES AND MOMENTS/37(TAS)
  "modulus "/1 -> FLAPPING DYNAMICS (TIP-PATH-PLANE APPROX)/7(g), AERODYNAMIC AND INERTIAL FORCES AND MOMENTS/8(g)
  Constant11/1 -> AERODYNAMIC AND INERTIAL FORCES AND MOMENTS/28(dyn_viscosity)
  Constant2/1 -> AERODYNAMIC AND INERTIAL FORCES AND MOMENTS/12(CHORD)
  Constant16/1 -> AERODYNAMIC AND INERTIAL FORCES AND MOMENTS/2(i_s)
  Constant1/1 -> AERODYNAMIC AND INERTIAL FORCES AND MOMENTS/10(ASLOPE)
  AERODYNAMIC AND INERTIAL FORCES AND MOMENTS/4(lambda) -> FLAPPING DYNAMICS (TIP-PATH-PLANE APPROX)/5(lambda)
  Gain/1 -> Mux/2  "a1"
  Constant22/1 -> AERODYNAMIC AND INERTIAL FORCES AND MOMENTS/6(EPSLN)
  Constant5/1 -> AERODYNAMIC AND INERTIAL FORCES AND MOMENTS/40(OMEGA)
  FLAPPING DYNAMICS (TIP-PATH-PLANE APPROX)/7(a0ddot) -> AERODYNAMIC AND INERTIAL FORCES AND MOMENTS/23(a0ddot)
  rho/1 -> AERODYNAMIC AND INERTIAL FORCES AND MOMENTS/36(rho)
  Constant3/1 -> AERODYNAMIC AND INERTIAL FORCES AND MOMENTS/13(CD)
  Constant/1 -> AERODYNAMIC AND INERTIAL FORCES AND MOMENTS/9(BLADES)
  AERODYNAMIC AND INERTIAL FORCES AND MOMENTS/2(Frotor) -> F_rotor/1
  Constant20/1 -> AERODYNAMIC AND INERTIAL FORCES AND MOMENTS/4(Jbeta)
  Theta0/1 -> FLAPPING DYNAMICS (TIP-PATH-PLANE APPROX)/3(Theta0), AERODYNAMIC AND INERTIAL FORCES AND MOMENTS/26(Theta0)
  Constant15/1 -> AERODYNAMIC AND INERTIAL FORCES AND MOMENTS/1(chi)
  Constant4/1 -> AERODYNAMIC AND INERTIAL FORCES AND MOMENTS/14(ROTOR)
  omega_TAS/1 -> AERODYNAMIC AND INERTIAL FORCES AND MOMENTS/38(omega_TAS), FLAPPING DYNAMICS (TIP-PATH-PLANE APPROX)/10(omega_TAS)
  Constant18/1 -> AERODYNAMIC AND INERTIAL FORCES AND MOMENTS/3(m_blade)
  Constant21/1 -> AERODYNAMIC AND INERTIAL FORCES AND MOMENTS/5(GAMMA)
  AERODYNAMIC AND INERTIAL FORCES AND MOMENTS/6(Q) -> Stop simulation if maximum transmission power rating is exceeded/1(Q)
  FLAPPING DYNAMICS (TIP-PATH-PLANE APPROX)/9(b1ddot) -> AERODYNAMIC AND INERTIAL FORCES AND MOMENTS/25(b1ddot)
  Constant12/1 -> AERODYNAMIC AND INERTIAL FORCES AND MOMENTS/29(k_ind)
  Constant8/1 -> AERODYNAMIC AND INERTIAL FORCES AND MOMENTS/30(STACG)
  AERODYNAMIC AND INERTIAL FORCES AND MOMENTS/5(T) -> To Workspace/1, Stop simulation if main rotor hub load limit is exceeded/1(T)
  FLAPPING DYNAMICS (TIP-PATH-PLANE APPROX)/1(a0) -> Gain2/1, AERODYNAMIC AND INERTIAL FORCES AND MOMENTS/17(a0)
  FLAPPING DYNAMICS (TIP-PATH-PLANE APPROX)/5(a1dot) -> AERODYNAMIC AND INERTIAL FORCES AND MOMENTS/21(a1dot)
  Constant6/1 -> AERODYNAMIC AND INERTIAL FORCES AND MOMENTS/33(STAH)
  AERODYNAMIC AND INERTIAL FORCES AND MOMENTS/3(lambda_i) -> FLAPPING DYNAMICS (TIP-PATH-PLANE APPROX)/4(lambda_i), lambda_i/1

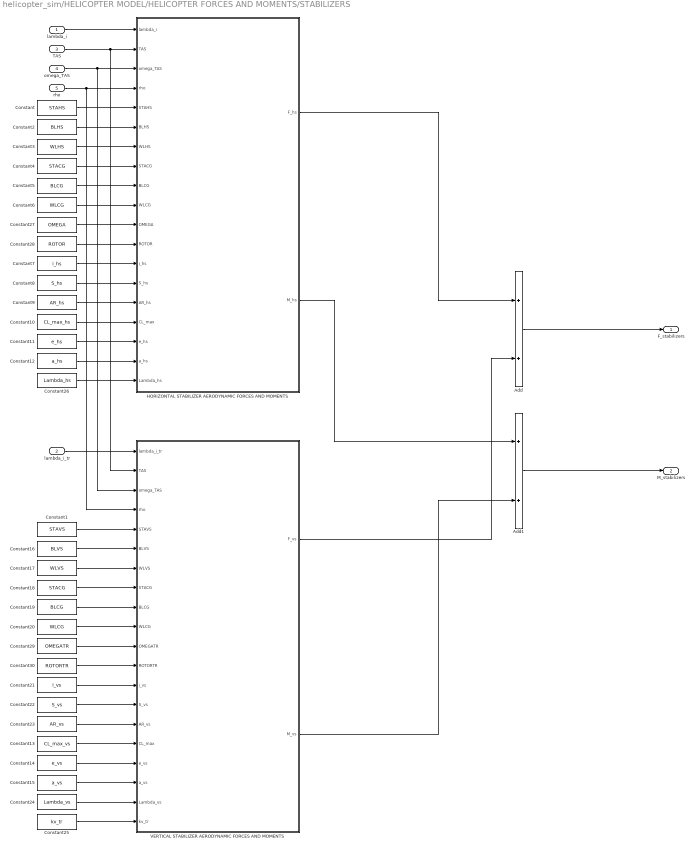
== system helicopter_sim/HELICOPTER MODEL/HELICOPTER FORCES AND MOMENTS/STABILIZERS  ==
  lambda_i : Inport
  lambda_i_tr : Inport  Port=2
  TAS : Inport  Port=3
  omega_TAS : Inport  Port=4
  rho : Inport  Port=5
  Add : Sum
  Add1 : Sum
  Constant : Constant  Value=STAHS
  Constant1 : Constant  Value=STAVS
  Constant10 : Constant  Value=CL_max_hs
  Constant11 : Constant  Value=e_hs
  Constant12 : Constant  Value=a_hs
  Constant13 : Constant  Value=CL_max_vs
  Constant14 : Constant  Value=e_vs
  Constant15 : Constant  Value=a_vs
  Constant16 : Constant  Value=BLVS
  Constant17 : Constant  Value=WLVS
  Constant18 : Constant  Value=STACG
  Constant19 : Constant  Value=BLCG
  Constant2 : Constant  Value=BLHS
  Constant20 : Constant  Value=WLCG
  Constant21 : Constant  Value=i_vs
  Constant22 : Constant  Value=S_vs
  Constant23 : Constant  Value=AR_vs
  Constant24 : Constant  Value=Lambda_vs
  Constant25 : Constant  Value=kv_tr
  Constant26 : Constant  Value=Lambda_hs
  Constant27 : Constant  Value=OMEGA
  Constant28 : Constant  Value=ROTOR
  Constant29 : Constant  Value=OMEGATR
  Constant3 : Constant  Value=WLHS
  Constant30 : Constant  Value=ROTORTR
  Constant4 : Constant  Value=STACG
  Constant5 : Constant  Value=BLCG
  Constant6 : Constant  Value=WLCG
  Constant7 : Constant  Value=i_hs
  Constant8 : Constant  Value=S_hs
  Constant9 : Constant  Value=AR_hs
  HORIZONTAL STABILIZER AERODYNAMIC FORCES AND MOMENTS : MATLAB Function  TreatAsAtomicUnit=on
  VERTICAL STABILIZER AERODYNAMIC FORCES AND MOMENTS : MATLAB Function  TreatAsAtomicUnit=on
  F_stabilizers : Outport
  M_stabilizers : Outport  Port=2
  wires:
  Constant28/1 -> HORIZONTAL STABILIZER AERODYNAMIC FORCES AND MOMENTS/12(ROTOR)
  Constant20/1 -> VERTICAL STABILIZER AERODYNAMIC FORCES AND MOMENTS/10(WLCG)
  HORIZONTAL STABILIZER AERODYNAMIC FORCES AND MOMENTS/1(F_hs) -> Add/1
  VERTICAL STABILIZER AERODYNAMIC FORCES AND MOMENTS/2(M_vs) -> Add1/2
  Constant5/1 -> HORIZONTAL STABILIZER AERODYNAMIC FORCES AND MOMENTS/9(BLCG)
  Constant19/1 -> VERTICAL STABILIZER AERODYNAMIC FORCES AND MOMENTS/9(BLCG)
  Constant14/1 -> VERTICAL STABILIZER AERODYNAMIC FORCES AND MOMENTS/17(e_vs)
  Constant4/1 -> HORIZONTAL STABILIZER AERODYNAMIC FORCES AND MOMENTS/8(STACG)
  Constant9/1 -> HORIZONTAL STABILIZER AERODYNAMIC FORCES AND MOMENTS/15(AR_hs)
  Constant6/1 -> HORIZONTAL STABILIZER AERODYNAMIC FORCES AND MOMENTS/10(WLCG)
  lambda_i_tr/1 -> VERTICAL STABILIZER AERODYNAMIC FORCES AND MOMENTS/1(lambda_i_tr)
  Constant27/1 -> HORIZONTAL STABILIZER AERODYNAMIC FORCES AND MOMENTS/11(OMEGA)
  Constant17/1 -> VERTICAL STABILIZER AERODYNAMIC FORCES AND MOMENTS/7(WLVS)
  HORIZONTAL STABILIZER AERODYNAMIC FORCES AND MOMENTS/2(M_hs) -> Add1/1
  Constant12/1 -> HORIZONTAL STABILIZER AERODYNAMIC FORCES AND MOMENTS/18(a_hs)
  Constant8/1 -> HORIZONTAL STABILIZER AERODYNAMIC FORCES AND MOMENTS/14(S_hs)
  Constant13/1 -> VERTICAL STABILIZER AERODYNAMIC FORCES AND MOMENTS/16(CL_max)
  Constant/1 -> HORIZONTAL STABILIZER AERODYNAMIC FORCES AND MOMENTS/5(STAHS)
  Constant15/1 -> VERTICAL STABILIZER AERODYNAMIC FORCES AND MOMENTS/18(a_vs)
  Constant30/1 -> VERTICAL STABILIZER AERODYNAMIC FORCES AND MOMENTS/12(ROTORTR)
  Constant2/1 -> HORIZONTAL STABILIZER AERODYNAMIC FORCES AND MOMENTS/6(BLHS)
  VERTICAL STABILIZER AERODYNAMIC FORCES AND MOMENTS/1(F_vs) -> Add/2
  Constant1/1 -> VERTICAL STABILIZER AERODYNAMIC FORCES AND MOMENTS/5(STAVS)
  Constant24/1 -> VERTICAL STABILIZER AERODYNAMIC FORCES AND MOMENTS/19(Lambda_vs)
  Constant23/1 -> VERTICAL STABILIZER AERODYNAMIC FORCES AND MOMENTS/15(AR_vs)
  Constant22/1 -> VERTICAL STABILIZER AERODYNAMIC FORCES AND MOMENTS/14(S_vs)
  Constant25/1 -> VERTICAL STABILIZER AERODYNAMIC FORCES AND MOMENTS/20(kv_tr)
  Constant11/1 -> HORIZONTAL STABILIZER AERODYNAMIC FORCES AND MOMENTS/17(e_hs)
  TAS/1 -> VERTICAL STABILIZER AERODYNAMIC FORCES AND MOMENTS/2(TAS), HORIZONTAL STABILIZER AERODYNAMIC FORCES AND MOMENTS/2(TAS)
  Constant21/1 -> VERTICAL STABILIZER AERODYNAMIC FORCES AND MOMENTS/13(i_vs)
  Constant3/1 -> HORIZONTAL STABILIZER AERODYNAMIC FORCES AND MOMENTS/7(WLHS)
  Constant26/1 -> HORIZONTAL STABILIZER AERODYNAMIC FORCES AND MOMENTS/19(Lambda_hs)
  Constant7/1 -> HORIZONTAL STABILIZER AERODYNAMIC FORCES AND MOMENTS/13(i_hs)
  Constant16/1 -> VERTICAL STABILIZER AERODYNAMIC FORCES AND MOMENTS/6(BLVS)
  Constant10/1 -> HORIZONTAL STABILIZER AERODYNAMIC FORCES AND MOMENTS/16(CL_max)
  rho/1 -> VERTICAL STABILIZER AERODYNAMIC FORCES AND MOMENTS/4(rho), HORIZONTAL STABILIZER AERODYNAMIC FORCES AND MOMENTS/4(rho)
  lambda_i/1 -> HORIZONTAL STABILIZER AERODYNAMIC FORCES AND MOMENTS/1(lambda_i)
  omega_TAS/1 -> VERTICAL STABILIZER AERODYNAMIC FORCES AND MOMENTS/3(omega_TAS), HORIZONTAL STABILIZER AERODYNAMIC FORCES AND MOMENTS/3(omega_TAS)
  Constant29/1 -> VERTICAL STABILIZER AERODYNAMIC FORCES AND MOMENTS/11(OMEGATR)
  Constant18/1 -> VERTICAL STABILIZER AERODYNAMIC FORCES AND MOMENTS/8(STACG)
  Add/1 -> F_stabilizers/1
  Add1/1 -> M_stabilizers/1

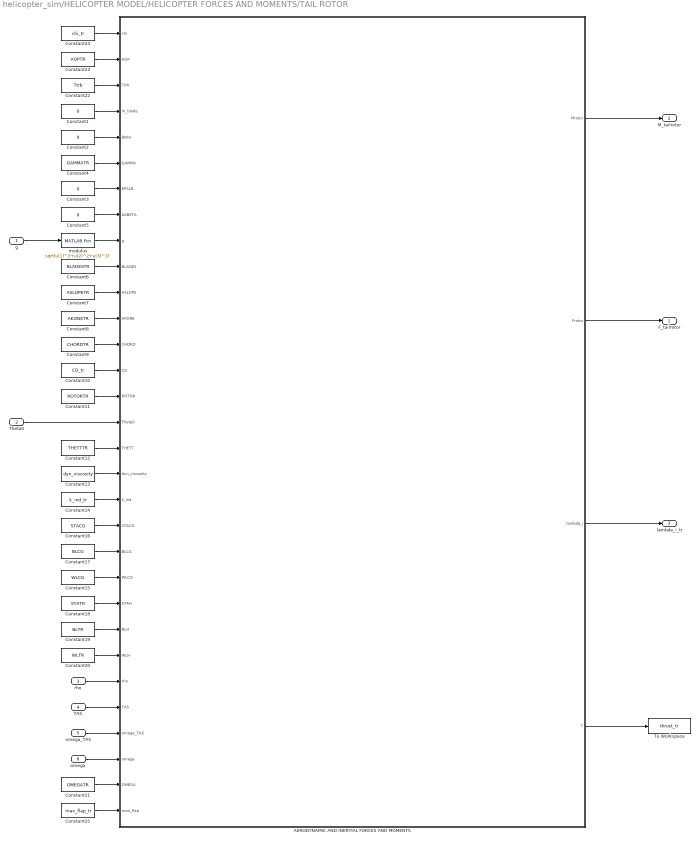
== system helicopter_sim/HELICOPTER MODEL/HELICOPTER FORCES AND MOMENTS/TAIL ROTOR  ==
  g : Inport
  Theta0 : Inport  Port=2
  rho : Inport  Port=3
  TAS : Inport  Port=4
  omega_TAS : Inport  Port=5
  omega : Inport  Port=6
  AERODYNAMIC AND INERTIAL FORCES AND MOMENTS : MATLAB Function  TreatAsAtomicUnit=on
  Constant{1..3,5} (4 alike) : Constant  Value=0
  Constant10 : Constant  Value=CD_tr
  Constant11 : Constant  Value=ROTORTR
  Constant12 : Constant  Value=THETTTR
  Constant13 : Constant  Value=dyn_viscosity
  Constant14 : Constant  Value=k_ind_tr
  Constant15 : Constant  Value=WLCG
  Constant16 : Constant  Value=STACG
  Constant17 : Constant  Value=BLCG
  Constant18 : Constant  Value=STATR
  Constant19 : Constant  Value=BLTR
  Constant20 : Constant  Value=WLTR
  Constant21 : Constant  Value=OMEGATR
  Constant22 : Constant  Value=Ttrb
  Constant23 : Constant  Value=AOPTR
  Constant24 : Constant  Value=chi_tr
  Constant25 : Constant  Value=max_flap_tr
  Constant4 : Constant  Value=GAMMATR
  Constant6 : Constant  Value=BLADESTR
  Constant7 : Constant  Value=ASLOPETR
  Constant8 : Constant  Value=AKONETR
  Constant9 : Constant  Value=CHORDTR
  To Workspace : ToWorkspace  VariableName=thrust_tr  SampleTime=-1
  "modulus " : MATLABFcn  MATLABFcn=sqrt(u(1)^2+u(2)^2+u(3)^2)
  F_tailrotor : Outport
  M_tailrotor : Outport  Port=2
  lambda_i_tr : Outport  Port=3
  wires:
  AERODYNAMIC AND INERTIAL FORCES AND MOMENTS/2(Frotor) -> F_tailrotor/1
  AERODYNAMIC AND INERTIAL FORCES AND MOMENTS/1(Mrotor) -> M_tailrotor/1
  Theta0/1 -> AERODYNAMIC AND INERTIAL FORCES AND MOMENTS/16(Theta0)
  Constant12/1 -> AERODYNAMIC AND INERTIAL FORCES AND MOMENTS/17(THETT)
  Constant8/1 -> AERODYNAMIC AND INERTIAL FORCES AND MOMENTS/12(AKONE)
  Constant21/1 -> AERODYNAMIC AND INERTIAL FORCES AND MOMENTS/30(OMEGA)
  Constant4/1 -> AERODYNAMIC AND INERTIAL FORCES AND MOMENTS/6(GAMMA)
  omega/1 -> AERODYNAMIC AND INERTIAL FORCES AND MOMENTS/29(omega)
  omega_TAS/1 -> AERODYNAMIC AND INERTIAL FORCES AND MOMENTS/28(omega_TAS)
  TAS/1 -> AERODYNAMIC AND INERTIAL FORCES AND MOMENTS/27(TAS)
  rho/1 -> AERODYNAMIC AND INERTIAL FORCES AND MOMENTS/26(rho)
  Constant20/1 -> AERODYNAMIC AND INERTIAL FORCES AND MOMENTS/25(WLH)
  Constant18/1 -> AERODYNAMIC AND INERTIAL FORCES AND MOMENTS/23(STAH)
  Constant19/1 -> AERODYNAMIC AND INERTIAL FORCES AND MOMENTS/24(BLH)
  Constant15/1 -> AERODYNAMIC AND INERTIAL FORCES AND MOMENTS/22(WLCG)
  Constant17/1 -> AERODYNAMIC AND INERTIAL FORCES AND MOMENTS/21(BLCG)
  Constant16/1 -> AERODYNAMIC AND INERTIAL FORCES AND MOMENTS/20(STACG)
  Constant14/1 -> AERODYNAMIC AND INERTIAL FORCES AND MOMENTS/19(k_ind)
  Constant13/1 -> AERODYNAMIC AND INERTIAL FORCES AND MOMENTS/18(dyn_viscosity)
  Constant11/1 -> AERODYNAMIC AND INERTIAL FORCES AND MOMENTS/15(ROTOR)
  Constant10/1 -> AERODYNAMIC AND INERTIAL FORCES AND MOMENTS/14(CD)
  Constant9/1 -> AERODYNAMIC AND INERTIAL FORCES AND MOMENTS/13(CHORD)
  Constant7/1 -> AERODYNAMIC AND INERTIAL FORCES AND MOMENTS/11(ASLOPE)
  Constant6/1 -> AERODYNAMIC AND INERTIAL FORCES AND MOMENTS/10(BLADES)
  "modulus "/1 -> AERODYNAMIC AND INERTIAL FORCES AND MOMENTS/9(g)
  g/1 -> "modulus "/1
  Constant5/1 -> AERODYNAMIC AND INERTIAL FORCES AND MOMENTS/8(AKBETA)
  Constant3/1 -> AERODYNAMIC AND INERTIAL FORCES AND MOMENTS/7(EPSLN)
  Constant1/1 -> AERODYNAMIC AND INERTIAL FORCES AND MOMENTS/4(m_blade)
  Constant2/1 -> AERODYNAMIC AND INERTIAL FORCES AND MOMENTS/5(Jbeta)
  Constant22/1 -> AERODYNAMIC AND INERTIAL FORCES AND MOMENTS/3(Ttrb)
  Constant23/1 -> AERODYNAMIC AND INERTIAL FORCES AND MOMENTS/2(AOP)
  AERODYNAMIC AND INERTIAL FORCES AND MOMENTS/3(lambda_i) -> lambda_i_tr/1
  Constant24/1 -> AERODYNAMIC AND INERTIAL FORCES AND MOMENTS/1(chi)
  Constant25/1 -> AERODYNAMIC AND INERTIAL FORCES AND MOMENTS/31(max_flap)
  AERODYNAMIC AND INERTIAL FORCES AND MOMENTS/4(T) -> To Workspace/1

== system helicopter_sim/HELICOPTER MODEL/trim-linearization routines/LINEARIZATION ==
  Bus Creator1 : BusCreator  Inputs=6
  Constant1 : Constant  Value=[0; 0; 0]
  Constant2 : Constant  Value=omega0
  Constant3 : Constant  Value=V0
  Constant4 : Constant  Value=euler0
  Constant5 : Constant  Value=[0; 0; 0]
  Constant6 : Constant  Value=Xe_0
  state : Outport
  wires:
  Constant5/1 -> Bus Creator1/5  "PQR_dot"
  Constant6/1 -> Bus Creator1/1  "NED"
  Constant4/1 -> Bus Creator1/2  "Euler"
  Constant3/1 -> Bus Creator1/3  "UVW"
  Constant2/1 -> Bus Creator1/4  "PQR"
  Bus Creator1/1 -> state/1
  Constant1/1 -> Bus Creator1/6  "UVW_dot"

== system helicopter_sim/HELICOPTER MODEL/trim-linearization routines/TRIM ==
  Bus Creator1 : BusCreator  Inputs=6
  Constant1 : Constant  Value=[0; 0; 0]
  Constant2 : Constant  Value=[0; 0; 0]
  Constant3 : Constant  Value=[0; 0; 0]
  Constant6 : Constant  Value=Xe_0
  Constant8 : Constant  Value=euler0
  Constant9 : Constant  Value=fc
  Matrix Multiply : Product  Multiplication=Matrix(*)
  Rotation Angles to Direction Cosine Matrix1 : Angle2Dcm  rotationOrder=XYZ
      settings: AttributesFormatString=Rotation Order: %<rotationOrder>
  state : Outport
  wires:
  Constant9/1 -> Matrix Multiply/2
  Bus Creator1/1 -> state/1
  Rotation Angles to Direction Cosine Matrix1/1 -> Matrix Multiply/1
  Constant6/1 -> Bus Creator1/1  "NED"
  Constant8/1 -> Rotation Angles to Direction Cosine Matrix1/1, Bus Creator1/2  "Euler"
  Matrix Multiply/1 -> Bus Creator1/3  "UVW"
  Constant1/1 -> Bus Creator1/4  "PQR"
  Constant2/1 -> Bus Creator1/5  "PQR_dot"
  Constant3/1 -> Bus Creator1/6  "UVW_dot"
